simulink model "Tut_Week_8_Sliding_Disturbance"  (R2020a)
settings: Solver=FixedStepAuto  StartTime=0.0  StopTime=10.0  FixedStep=0.001  RelTol=1e-3
libraries: simulink x1
settings Model: Creator=김태욱  LastModifiedBy=skim
settings SolverCC: ZeroCrossAlgorithm=Adaptive
settings DebuggingCC: IgnoredZcDiagnostic=none

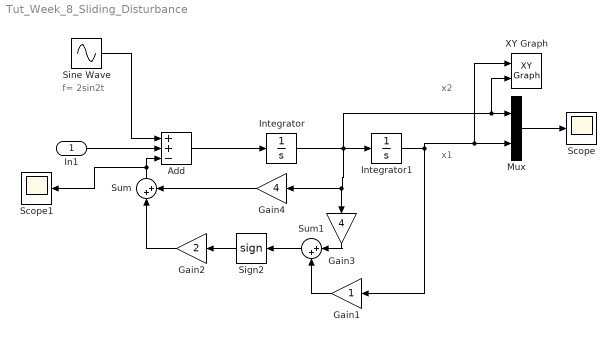
== system Tut_Week_8_Sliding_Disturbance ==
  note: f= 2sin2t
  note: x1
  note: x2
  In1 : Inport
  Add : Sum  Inputs=++-
  Gain1 : Gain
  Gain2 : Gain  Gain=2
  Gain3 : Gain  Gain=4
  Gain4 : Gain  Gain=4
  Integrator : Integrator  InitialCondition=0.5
  Integrator1 : Integrator  InitialCondition=0.5
  Mux : Mux  Inputs=2
  Scope : Scope
  Scope1 : Scope
  Sign2 : Signum
  Sine Wave : Sin  Amplitude=2  Frequency=2  SampleTime=0
  Sum : Sum  Inputs=|++
  Sum1 : Sum  Inputs=|++
  XY Graph : simulink/Sinks/XY Graph  xmin=-1  xmax=1  ymin=-1  ymax=1  st=-1
  wires:
  Gain4/1 -> Sum/2
  Integrator/1 -> XY Graph/2, Mux/1, Gain4/1, Gain3/1, Integrator1/1
  Mux/1 -> Scope/1
  Integrator1/1 -> Gain1/1, XY Graph/1, Mux/2
  Sine Wave/1 -> Add/1
  Sum/1 -> Add/3, Scope1/1
  Add/1 -> Integrator/1
  In1/1 -> Add/2
  Gain1/1 -> Sum1/2
  Sum1/1 -> Sign2/1
  Sign2/1 -> Gain2/1
  Gain2/1 -> Sum/1
  Gain3/1 -> Sum1/1
